simulink model "PS_Simulation_Modes"  (R2013b)
settings: Solver=ode23tb  SolverMode=SingleTasking  StartTime=0.0  StopTime=0.2  RelTol=1e-4
libraries: powerlib x15, powerlib_meascontrol x1
Description:
  | Copyright 2008-2013 The MathWorks, Inc.
settings Model: ExtModeTrigMode=oneshot  ExtModeArmWhenConnect=off  ExtModeAutoUpdateStatusClock=off  Creator=MathWorks  LastModifiedBy=smiller
settings SolverCC: ZeroCrossAlgorithm=Adaptive
settings DataIOCC: LimitDataPoints=off  SignalLoggingSaveFormat=ModelDataLogs  SignalLoggingName=sigsOut
settings OptimizationCC: BlockReduction=off  BooleanDataType=off  ExpressionDepthLimit=2147483647  InitFltsAndDblsToZero=on  EfficientMapNaN2IntZero=off
settings DebuggingCC: SaveWithParameterizedLinksMsg=none  CheckExecutionContextPreStartOutputMsg=on  CheckExecutionContextRuntimeOutputMsg=on  SignalResolutionControl=TryResolveAllWithWarning  SolverPrmCheckMsg=none  MultiTaskDSMMsg=warning  MultiTaskCondExecSysMsg=none  SigSpecEnsureSampleTimeMsg=none  FcnCallInpInsideContextMsg=UseLocalSettings  StateNameClashWarn=warning
settings HardwareCC: TargetUnknown=on
settings RTWCC: IncludeERTFirstTime=on
settings GRTTargetCC: TargetFcnLib=ansi_tfl_tmw.mat  CombineOutputUpdateFcns=off  GRTInterface=on

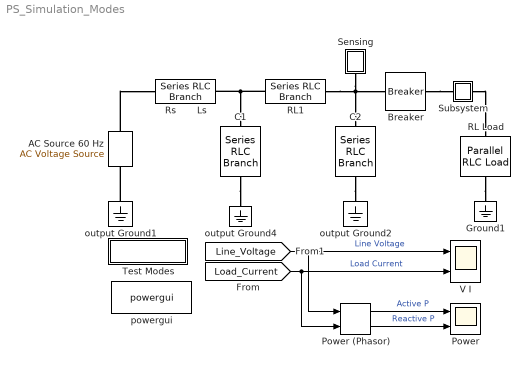
== system PS_Simulation_Modes ==
  AC Source 60 Hz : powerlib/Electrical Sources/AC Voltage Source  Description=source block  Amplitude=230e3/sqrt(3)*sqrt(2)  Phase=90  Frequency=60  SampleTime=0  Measurements=None
      settings: AttributesFormatString=\n
  Breaker : powerlib/Elements/Breaker  BreakerResistance=0.01  InitialState=1  SnubberResistance=inf  SnubberCapacitance=0  SwitchingTimes="[ 2/60  7/60 ]"  External=off  Measurements=None  MoreParameters=off  NoBreakLoop=off
      settings: AttributesFormatString=\n
  C1 : powerlib/Elements/Series RLC Branch  LConnTagsString=__new0  RConnTagsString=__new0  BranchType=C  Resistance=[]  Inductance=[]  SetiL0=off  InitialCurrent=0  Capacitance=0.967e-06  Setx0=off  InitialVoltage=0  Measurements=None
  C2 : powerlib/Elements/Series RLC Branch  LConnTagsString=__new0  RConnTagsString=__new0  BranchType=C  Resistance=[]  Inductance=[]  SetiL0=off  InitialCurrent=0  Capacitance=0.967e-06  Setx0=off  InitialVoltage=0  Measurements=None
  Ground1 : powerlib/Elements/Ground  LConnTagsString=a
  Power : Scope  NumInputPorts=2
      settings: TimeRange=0.2  YMin=0~-1  YMax=80000000~1  SaveName=VI_Data1
  Power (Phasor) : powerlib_meascontrol/Measurements/Power (Phasor)
  RL Load : powerlib/Elements/Parallel RLC Load  LConnTagsString=a  RConnTagsString=__new0  NominalVoltage=132.8e3  NominalFrequency=60  ActivePower=75e6  InductivePower=20e6  CapacitivePower=0  Setx0=off  InitialVoltage=0  SetiL0=off  InitialCurrent=0  Measurements=None
      settings: AttributesFormatString=\n
  RL1 : powerlib/Elements/Series RLC Branch  LConnTagsString=__new0  RConnTagsString=__new0  BranchType=RL  Resistance=5.2  Inductance=138e-3  SetiL0=off  InitialCurrent=0  Capacitance=[]  Setx0=off  InitialVoltage=0  Measurements=None
  Rs       Ls : powerlib/Elements/Series RLC Branch  LConnTagsString=__new0  RConnTagsString=__new0  BranchType=RL  Resistance=2.645  Inductance=70.2e-03  SetiL0=off  InitialCurrent=0  Capacitance=[]  Setx0=off  InitialVoltage=0  Measurements=None
  Sensing : Subsystem
      mask Display: disp('v');
  Subsystem : Subsystem
      mask Display: disp('i');
  Test Modes : Subsystem
      settings: OpenFcn=PS_Simulation_Modes_Test
      mask Display: disp('Test Modes');
  V I : Scope  NumInputPorts=2
      settings: TimeRange=0.2  YMin=-400000~-1000  YMax=400000~1000  SaveName=VI_Data
  output Ground1 : powerlib/Elements/Ground  LConnTagsString=a
  output Ground2 : powerlib/Elements/Ground  LConnTagsString=a
  output Ground4 : powerlib/Elements/Ground  LConnTagsString=a
  powergui : powerlib/powergui  Priority=2  SimulationMode=Continuous  SolverType=Tustin  SampleTime=1e-4  frequency=60  SPID=off  DisableSnubberDevices=off  DisableRonSwitches=off  DisableVfSwitches=off  SwTol=0  Interpol=off  DisplayEquations=off  frequencyindice=60  Pbase=100e6  ErrMax=1e-4  Iterations=50  UnitsV=kV  UnitsW=MW  FunctionMessages=off  echomessages=off  HookPort=off  EnableUseOfTLC=off  x0status=blocks  RestoreLinks=warning  ResistiveCurrentMeasurement=off  Frange=logspace(0,3,50)  Ylog=off  Xlog=off  ShowGrid=off  save=off  variable=ZData  ZoomFFT=on  StartTime=0.0  cycles=1  DisplayStyle=off  fundamental=60  FreqAxis=off  MaxFrequency=1000  frequencyindicesteady=1  RmsSteady=1  display=off  Ts=0  methode=off
  wires:
  [Line_Voltage] -> V I/1, Power (Phasor)/1  "Line Voltage"
  [Load_Current] -> V I/2, Power (Phasor)/2  "Load Current"
  Power (Phasor)/1 -> Power/1  "Active P"
  Power (Phasor)/2 -> Power/2  "Reactive P"
  connections:
  RL Load/RConn1 -- Ground1/LConn1
  AC Source 60 Hz/RConn1 -- Rs       Ls/LConn1
  output Ground1/LConn1 -- AC Source 60 Hz/LConn1
  RL1/LConn1 -- Rs       Ls/RConn1 -- C1/LConn1
  C1/RConn1 -- output Ground4/LConn1
  C2/RConn1 -- output Ground2/LConn1
  RL1/RConn1 -- Sensing/RConn1 -- Breaker/LConn1 -- C2/LConn1
  Breaker/RConn1 -- Subsystem/LConn1
  Subsystem/RConn1 -- RL Load/LConn1

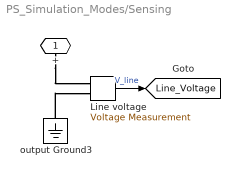
== system PS_Simulation_Modes/Sensing ==
  Line voltage : powerlib/Measurements/Voltage Measurement  Tag=PoWeRsYsTeMmEaSuReMeNt  PhasorSimulation=off  OutputType=Magnitude  PSBequivalent=0
  output Ground3 : powerlib/Elements/Ground  LConnTagsString=a
  + : PMIOPort  Port=1  Side=Right
  tag scope: Line_Voltage=global
  wires:
  Line voltage/1 -> [Line_Voltage]  "V_line"
  connections:
  output Ground3/LConn1 -- Line voltage/LConn2
  +/RConn1 -- Line voltage/LConn1

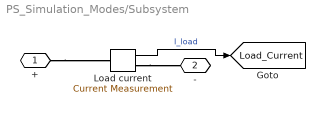
== system PS_Simulation_Modes/Subsystem ==
  Load current : powerlib/Measurements/Current Measurement  Tag=PoWeRsYsTeMmEaSuReMeNt  PhasorSimulation=off  OutputType=Magnitude  PSBequivalent=0
  + : PMIOPort  Port=1  Side=Left
  - : PMIOPort  Port=2  Side=Right
  tag scope: Load_Current=global
  wires:
  Load current/1 -> [Load_Current]  "I_load"
  connections:
  +/RConn1 -- Load current/LConn1
  Load current/RConn1 -- -/RConn1

== system PS_Simulation_Modes/Test Modes ==
